simulink model "Core_Model_Controlled"  (R2023a)
settings: Solver=FixedStepAuto  StartTime=0.0  StopTime=Z  FixedStep=1/24  RelTol=1e-3
values from neighbouring files (symbols this model uses):
  c_eh = 0.85    [Model_Parameters.m]
  C_g = 1    [Model_Parameters.m]
  cc_e = -0.85    [Model_Parameters.m]
  id_a = 0.8*0.028*1.2    (= 0.02688)    [Model_Parameters.m]
  id_g = 0.8*0.072*1.2    (= 0.06912)    [Model_Parameters.m]
  id_l = 0.4*0.139*1.2    (= 0.06672)    [Model_Parameters.m]
  id_r = 0.4*0.428*1.2    (= 0.20544)    [Model_Parameters.m]
  id_z = 0.4*0.33*1.2    (= 0.1584)    [Model_Parameters.m]
  L_a = 0.25    [Model_Parameters.m]
  L_g = 0.1    [Model_Parameters.m]
  L_l = 0.2    [Model_Parameters.m]
  L_r = 0.05    [Model_Parameters.m]
  L_z = 0.08    [Model_Parameters.m]
  R_H2 = 0.05    [Model_Parameters.m]
  R_lh = 0.025    [Model_Parameters.m]
  R_ng = 0.025    [Model_Parameters.m]
  SF_MWh = SF_GWh*1e3    [Main_Script.m]
libraries: fl_lib x120, nesl_utility x93, ee_lib x36, slpidlib x1
(part 1 of 3)
settings Model: Creator=pienv  LastModifiedBy=pienv

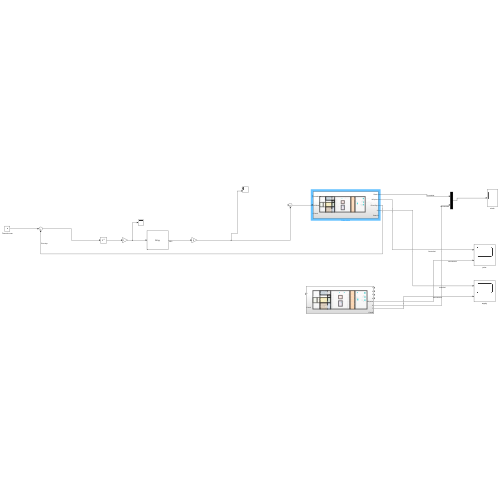
[thumbnail: Simulink's stored preview of the top-level diagram]
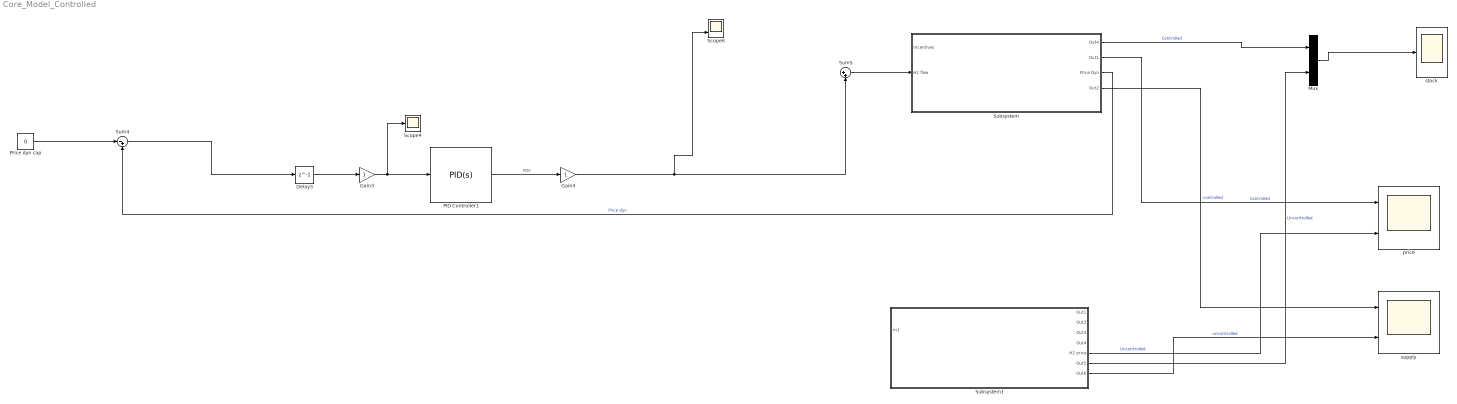
== system Core_Model_Controlled ==
  Delay3 : Delay  DelayLength=1
  Gain3 : Gain
  Gain4 : Gain
  Mux : Mux  Inputs=2
  PID Controller1 : slpidlib/PID Controller  Controller=PID  Form=Parallel  TimeDomain=Continuous-time  UseExternalTs=off  SampleTime=1/24  IntegratorMethod=Forward Euler  FilterMethod=Forward Euler  ControllerParametersSource=internal  P=20  I=4  UseKiTs=off  D=10  N=1  UseFilter=on  TunerSelectOption=Transfer Function Based (PID Tuner App)  InitialConditionSource=internal  InitialConditionForIntegrator=0  InitialConditionForFilter=0  DifferentiatorICPrevScaledInput=0  ExternalReset=none  TrackingMode=off  Kt=1  LimitOutput=off  SatLimitsSource=internal  UpperSaturationLimit=inf  LowerSaturationLimit=-inf  LinearizeAsGain=on  AntiWindupMode=none  Kb=1  LimitIntegrator=off  UpperIntegratorSaturationLimit=inf  LowerIntegratorSaturationLimit=-inf  POutMin=[]  POutMax=[]  IOutMin=[]  IOutMax=[]  DOutMin=[]  DOutMax=[]  NOutMin=[]  NOutMax=[]  SumOutMin=[]  SumOutMax=[]  SaturationOutMin=[]  SaturationOutMax=[]  PParamMin=[]  PParamMax=[]  IParamMin=[]  IParamMax=[]  DParamMin=[]  DParamMax=[]  NParamMin=[]  NParamMax=[]  KbParamMin=[]  KbParamMax=[]  KtParamMin=[]  KtParamMax=[]  KbOutMin=[]  KbOutMax=[]  KtOutMin=[]  KtOutMax=[]  IntegratorOutMin=[]  IntegratorOutMax=[]  FilterOutMin=[]  FilterOutMax=[]  SumI1OutMin=[]  SumI1OutMax=[]  SumI2OutMin=[]  SumI2OutMax=[]  SumI3OutMin=[]  SumI3OutMax=[]  SumI4OutMin=[]  SumI4OutMax=[]  SumDOutMin=[]  SumDOutMax=[]  DifferentiatorOutMin=[]  DifferentiatorOutMax=[]  FilterDiffOutCoefMin=[]  FilterDiffOutCoefMax=[]  ReciprocalOutMin=[]  ReciprocalOutMax=[]  SumDenOutMin=[]  SumDenOutMax=[]  SumNumOutMin=[]  SumNumOutMax=[]  DivideOutMin=[]  DivideOutMax=[]  UdiffTsProdOutMin=[]  UdiffTsProdOutMax=[]  NTsProdOutMin=[]  NTsProdOutMax=[]  UintegralTsProdOutMin=[]  UintegralTsProdOutMax=[]  UngainTsProdOutMin=[]  UngainTsProdOutMax=[]  ClampingZeroOutDataTypeStr=Inherit: Inherit via back propagation  ClampingZeroOutMin=[]  ClampingZeroOutMax=[]  FilterDenConstantOutDataTypeStr=Inherit: Inherit via back propagation  FilterDenConstantOutMin=[]  FilterDenConstantOutMax=[]  PCopyOutDataTypeStr=Inherit: Inherit via back propagation  PCopyOutMin=[]  PCopyOutMax=[]  NCopyOutDataTypeStr=Inherit: Inherit via back propagation  NCopyOutMin=[]  NCopyOutMax=[]  IntegratorContinuousStateAttributes=''  IntegratorStateMustResolveToSignalObject=off  IntegratorRTWStateStorageClass=Auto  FilterContinuousStateAttributes=''  FilterStateMustResolveToSignalObject=off  FilterRTWStateStorageClass=Auto  ParallelPVariant=InternalParameters  IdealPVariant=Disabled  IVariant=InternalParameters  DVariant=InternalParameters  IntegratorVariant=Continuous  SatVariant=Disabled  AWVariant=Passthrough  PCopyVariant=Disabled  TRVariant=Disabled  FdbkBlocksVariant=Forward  IdealPFdbkVariant=Disabled  SatFdbkVariant=Disabled  DerivativeFilterVariant=ContFilter  NVariant=InternalParameters  NCopyVariant=Disabled  FilterICVariant=InternalICsFilter  IntegratorICVariant=InternalICs  ExternalResetVariant=Disabled  TRSumVariant=Passthrough  SumFdbkVariant=Disabled  SumVariant=Sum_PID  TsampFilterVariant=InternalTs  TsampNgainVariant=Passthrough  TsampIntegralVariant=Disabled_SignalSpec  ExternalSaturationOutDataTypeStr=Inherit: Same as second input
  Price dyn cap : Constant  Value=0
  Scope4 : Scope
  Scope6 : Scope  NumInputPorts=2
  Subsystem : Subsystem
  Subsystem1 : Subsystem
  Sum4 : Sum  Inputs=|-+
  Sum5 : Sum  Inputs=|++
  price : Scope  NumInputPorts=2
  stock : Scope
  supply : Scope  NumInputPorts=2
  wires:
  Subsystem/2(Out1) -> price/1  "Controlled"
  Mux/1 -> stock/1
  Subsystem/1(Out4) -> Mux/1  "Controlled"
  Price dyn cap/1 -> Sum4/1
  Gain3/1 -> Scope4/1, PID Controller1/1
  Delay3/1 -> Gain3/1
  Sum4/1 -> Delay3/1
  PID Controller1/1 -> Gain4/1  "PDC"
  Subsystem/3(Price Dyn) -> Sum4/2  "Price dyn"
  Sum5/1 -> Subsystem/2(H2 flow)
  Gain4/1 -> Scope6/2, Sum5/2
  Subsystem1/5(H2 price) -> price/2  "Uncontrolled"
  Subsystem1/6(Out5) -> Mux/2  "Uncontrolled"
  Subsystem1/7(Out6) -> supply/2  "uncontrolled"
  Subsystem/4(Out2) -> supply/1  "controlled"

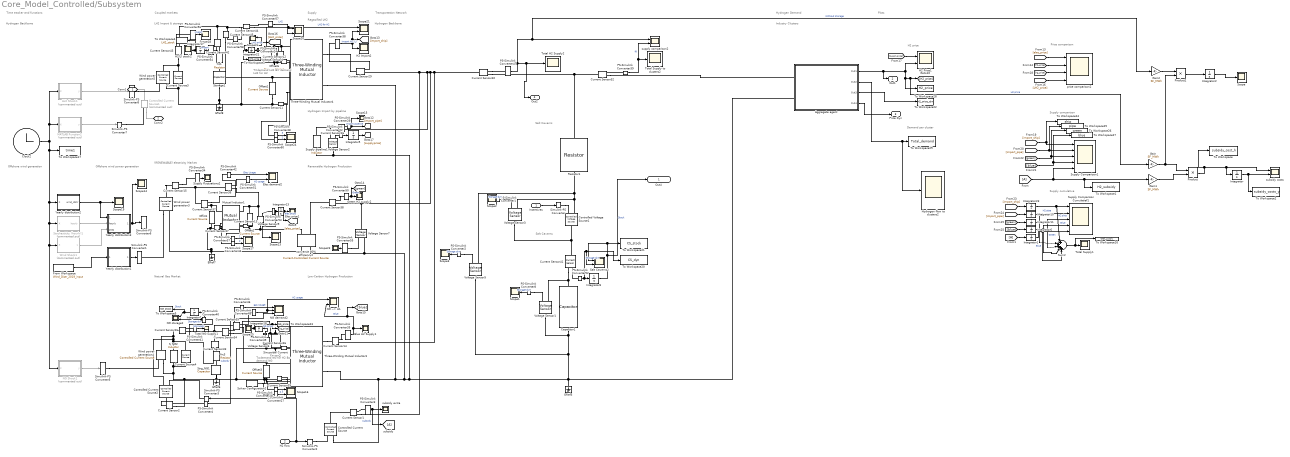
== system Core_Model_Controlled/Subsystem ==
  note: H2 price
  note: Supply cumulative
  note: Demand per cluster
  note: Renewable Hydrogen Production
  note: Offshore wind generation
  note: Hydrogen Import by pipeline
  note: Time tracker and functions
  note: Regasified LH2
  note: Hydrogen Backbone
  note: Hydrogen Backbone
  note: Coupled markets
  note: Supply comparison
  note: Salt Caverns
  note: Price comparison
  note: Transportation Network
  note: Plots
  note: Industry Clusters
  note: Hydrogen Demand
  note: Low-Carbon Hydrogen Production
  note: LH2 Import & storage
  note: T=demand LH2
      | B= demand LH2 for H2
  note: (RENEWABLE) electricity Market
  note: T=demand NG for H2
      | B= demand NG
  note: Supply
  note: Salt Caverns
  note: Offshore wind power generation
  note: Natural Gas Market
  Incentives : Inport
  H2 flow : Inport  Port=2
  Aggregate agent : Subsystem
  Blue H2 Supply1 : Scope
  Capacitor1 : fl_lib/Electrical/Electrical Elements/Capacitor  c=C_sc F  r=0 Ohm  g=0 1/Ohm  i_specify=on  i_priority=None  i=0.1 A  i_nominal_specify=off  i_nominal_unit=A  i_nominal_value=0.1  v_specify=off  v_priority=None  v=0 V  v_nominal_specify=off  v_nominal_unit=V  v_nominal_value=1  vc_specify=off  vc_priority=High  vc=0 V  vc_nominal_specify=off  vc_nominal_unit=V  vc_nominal_value=1
  Clock2 : Clock
      settings: Decimation=24
  Controlled Current Source : fl_lib/Electrical/Electrical Sources/Controlled Current Source
  Controlled Current Source1 : fl_lib/Electrical/Electrical Sources/Controlled Current Source  Commented=on
  Controlled Current Source2 : fl_lib/Electrical/Electrical Sources/Controlled Current Source
  Controlled Voltage Source1 : fl_lib/Electrical/Electrical Sources/Controlled Voltage Source
  Current Sensor{1..2,11..16,26,29,32..47} (26 alike) : fl_lib/Electrical/Electrical Sensors/Current Sensor
  Current Source3 : ee_lib/Sources/Current Source  dc_current=I_LH2 A  ac_current=0 A  ac_shift=0 rad  ac_frequency=60 Hz  noise_mode=ee.enum.sources.noise.Disabled  PSD=0 A^2/Hz  sample_time=1e-3 s  repeatability=ee.enum.sources.repeatability.NotRepeatable  user_seed=0  auto_seed=3890346746  i_specify=off  i_priority=None  i=0 A  i_nominal_specify=off  i_nominal_unit=A  i_nominal_value=1  v_specify=off  v_priority=None  v=0 V  v_nominal_specify=off  v_nominal_unit=V  v_nominal_value=1
  Current Source4 : ee_lib/Sources/Current Source  dc_current=v_sng A  ac_current=0 A  ac_shift=0 rad  ac_frequency=60 Hz  noise_mode=ee.enum.sources.noise.Disabled  PSD=0 A^2/Hz  sample_time=1e-3 s  repeatability=ee.enum.sources.repeatability.NotRepeatable  user_seed=0  auto_seed=545404223  i_specify=off  i_priority=None  i=0 A  i_nominal_specify=off  i_nominal_unit=A  i_nominal_value=1  v_specify=off  v_priority=None  v=0 V  v_nominal_specify=off  v_nominal_unit=V  v_nominal_value=1
  ERef{5..8} (4 alike) : fl_lib/Electrical/Electrical Elements/Electrical Reference
  Elec demand2 : Scope  NumInputPorts=2
  Elec price1 : Scope
  From : From
  From Workspace : FromWorkspace  VariableName=Wind_Distr_2019_input  OutDataTypeStr=double
  From1 : From
  Gain : Gain  Gain=SF_MWh
  Gain1 : Gain  Gain=SF_MWh
  Gain2 : Gain  Gain=SF_MWh
  Green H2 supply2 : Scope
  H2 Import2 : Scope
  H2 Price1 : Scope  NumInputPorts=2
  H2(L) stock2 : Scope
  Hydrogen flow to clusters2 : Scope
  Integrator{,1..2,5..8,10..11,13,17..18,21,23} (14 alike) : Integrator
  LH2 Shock1 : MATLAB Function  Commented=on  TreatAsAtomicUnit=on
  MATLAB Function2 : MATLAB Function  Commented=on  TreatAsAtomicUnit=on
  Mutual Inductor1 : fl_lib/Electrical/Electrical Elements/Mutual Inductor  L1=L_eh H  L2=L_e H  k=cc_e  i1_specify=off  i1_priority=High  i1=0 A  i1_nominal_specify=off  i1_nominal_unit=A  i1_nominal_value=1  i2_specify=off  i2_priority=High  i2=0 A  i2_nominal_specify=off  i2_nominal_unit=A  i2_nominal_value=1  v1_specify=off  v1_priority=None  v1=0 V  v1_nominal_specify=off  v1_nominal_unit=V  v1_nominal_value=1  v2_specify=off  v2_priority=None  v2=0 V  v2_nominal_specify=off  v2_nominal_unit=V  v2_nominal_value=1
      settings: InternalSimscapePortConfiguration="{\"Bottom\":[],\"Left\":[{\"id\":\"p1\",\"label\":\"1+\",\"type\":\"foundation.electrical.electrical\"},{\"id\":\"n1\",\"label\":\"1-\",\"type\":\"foundation.electrical.electrical\"}],\"Right\":[{\"id\":\"p2\",\"label\":\"2+\",\"type\":\"foundation.electrical.electrical\"},{\"id\":\"n2\",\"label\":\"2-\",\"type\":\"foundation.electrical.electrical\"}],\"Top\":[]}"
  NG --> H1 : Scope  NumInputPorts=2
  NG Shock1 : MATLAB Function  Commented=on  TreatAsAtomicUnit=on
  NG demand2 : Scope  NumInputPorts=3
  NG storage2 : Scope  NumInputPorts=2
  Offset1 : ee_lib/Sources/Current Source  dc_current=id_lh2h A  ac_current=0 A  ac_shift=0 rad  ac_frequency=0 Hz  noise_mode=0  PSD=0 A^2/Hz  sample_time=1e-3 s  repeatability=1  user_seed=0  auto_seed=3922919431  i_specify=off  i_priority=None  i=0 A  i_nominal_specify=off  i_nominal_unit=A  i_nominal_value=1  v_specify=off  v_priority=None  v=0 V  v_nominal_specify=off  v_nominal_unit=V  v_nominal_value=1
  Offset2 : ee_lib/Sources/Current Source  dc_current=id_eh A  ac_current=0 A  ac_shift=0 rad  ac_frequency=0 Hz  noise_mode=0  PSD=0 A^2/Hz  sample_time=1e-3 s  repeatability=1  user_seed=0  auto_seed=2715962282  i_specify=off  i_priority=None  i=0 A  i_nominal_specify=off  i_nominal_unit=A  i_nominal_value=1  v_specify=off  v_priority=None  v=0 V  v_nominal_specify=off  v_nominal_unit=V  v_nominal_value=1
  Offset3 : ee_lib/Sources/Current Source  dc_current=id_ngh A  ac_current=0 A  ac_shift=0 rad  ac_frequency=0 Hz  noise_mode=0  PSD=0 A^2/Hz  sample_time=1e-3 s  repeatability=1  user_seed=0  auto_seed=418932850  i_specify=off  i_priority=None  i=0 A  i_nominal_specify=off  i_nominal_unit=A  i_nominal_value=1  v_specify=off  v_priority=None  v=0 V  v_nominal_specify=off  v_nominal_unit=V  v_nominal_value=1
  Offset6 : ee_lib/Sources/Current Source  dc_current=id_lh2 A  ac_current=0 A  ac_shift=0 rad  ac_frequency=0 Hz  noise_mode=0  PSD=0 A^2/Hz  sample_time=1e-3 s  repeatability=1  user_seed=0  auto_seed=1196140742  i_specify=off  i_priority=None  i=0 A  i_nominal_specify=off  i_nominal_unit=A  i_nominal_value=1  v_specify=off  v_priority=None  v=0 V  v_nominal_specify=off  v_nominal_unit=V  v_nominal_value=1
  Offst1 : ee_lib/Sources/Current Source  dc_current=id_e A  ac_current=0 A  ac_shift=0 rad  ac_frequency=0 Hz  noise_mode=0  PSD=0 A^2/Hz  sample_time=1e-3 s  repeatability=1  user_seed=0  auto_seed=2348838240  i_specify=off  i_priority=None  i=0 A  i_nominal_specify=off  i_nominal_unit=A  i_nominal_value=1  v_specify=off  v_priority=None  v=0 V  v_nominal_specify=off  v_nominal_unit=V  v_nominal_value=1
  PS-Simulink Converter{1..4,8,22,24,27..29,34..35,37..42,44..56,60} (32 alike) : nesl_utility/PS-Simulink Converter  PhysicalDomain=network_engine_domain  SubClassName=ps_output  LeftPortType=input  RightPortType=output  PseudoPeriodic=off  Frequencies=[]  VectorFormat=1-D array  Unit=1  AffineConversion=off
  PS-Simulink Converter57 : nesl_utility/PS-Simulink Converter  PhysicalDomain=network_engine_domain  SubClassName=ps_output  LeftPortType=input  RightPortType=output  PseudoPeriodic=off  Frequencies=[]  VectorFormat=inherit  Unit=inherit  AffineConversion=off
  PS-Simulink Converter58 : nesl_utility/PS-Simulink Converter  PhysicalDomain=network_engine_domain  SubClassName=ps_output  LeftPortType=input  RightPortType=output  PseudoPeriodic=off  Frequencies=[]  VectorFormat=inherit  Unit=inherit  AffineConversion=off
  Product : Product
  Product1 : Product
  Resistor1 : fl_lib/Electrical/Electrical Elements/Resistor  R=R_H2 Ohm  i_specify=off  i_priority=None  i=0 A  i_nominal_specify=off  i_nominal_unit=A  i_nominal_value=1  v_specify=off  v_priority=None  v=0 V  v_nominal_specify=off  v_nominal_unit=V  v_nominal_value=1
  S_NG2 : ee_lib/Passive/Inductor  l=L_sng H  enable_L_tol=ee.enum.toleranceApplication.none  L_tol=20  tol_distribution=ee.enum.toleranceDistribution.uniform  nSigma=4  r=0 Ohm  g=0 1/Ohm  enable_operating_limits=ee.enum.enable.no  operating_limit_action=ee.enum.passive.reportOpLim.warn  max_working_current=1 A  power_rating=1 W  enable_faults=ee.enum.enable.no  fault_action=simscape.enum.assert.action.none  lambdaPercent=50  k_faulted=0.9999  turnsShort=ee.enum.passive.inductor.turnsShortOption.no  openCct=ee.enum.enable.no  groundShort=ee.enum.passive.inductor.groundShortOption.no  groundShortG=0 1/Ohm  tau_fault=1e-3 s  fault_trigger=ee.enum.faults.faultTrigger.temporal  t_fault=1 s  max_permissible_voltage=100 V  n_fail_on_voltage=1  max_permissible_current=1 A  t_fail_on_current=1 s  i_L_specify=off  i_L_priority=High  i_L=0 A  i_L_nominal_specify=off  i_L_nominal_unit=A  i_L_nominal_value=1
  Salt Caverns2 : Scope  NumInputPorts=2
  Scope{,1..3,13..15,18..19,23,25} (11 alike) : Scope
  Scope{16..17,20..22,24} (6 alike) : Scope  NumInputPorts=2
  Simulink-PS Converter{,2..3,5,7..8} (6 alike) : nesl_utility/Simulink-PS Converter  PhysicalDomain=network_engine_domain  SubClassName=ps_input  LeftPortType=input  RightPortType=output  PseudoPeriodic=off  Frequencies=[]  NoiseDistribution=none  NoiseParameters=[]  Unit=1  AffineConversion=off  FilteringAndDerivatives=provide  SimscapeFilterOrder=1  InputFilterTimeConstant=0.001  UdotUserProvided=0
  Simulink-PS Converter1 : nesl_utility/Simulink-PS Converter  PhysicalDomain=network_engine_domain  SubClassName=ps_input  LeftPortType=input  RightPortType=output  PseudoPeriodic=off  Frequencies=[]  NoiseDistribution=none  NoiseParameters=[]  Unit=1  AffineConversion=off  FilteringAndDerivatives=filter  SimscapeFilterOrder=2  InputFilterTimeConstant=0.001  UdotUserProvided=0
  Simulink-PS Converter6 : nesl_utility/Simulink-PS Converter  PhysicalDomain=network_engine_domain  SubClassName=ps_input  LeftPortType=input  RightPortType=output  PseudoPeriodic=off  Frequencies=[]  NoiseDistribution=none  NoiseParameters=[]  Unit=1  AffineConversion=off  FilteringAndDerivatives=filter  SimscapeFilterOrder=2  InputFilterTimeConstant=0.001  UdotUserProvided=0
  Sinusoidal Current Source2 : ee_lib/Additional Components/SPICE Sources/Sinusoidal Current Source  IO=id_ng_IO A  IA=id_ng_IA A  FREQ=id_ng_FREQ Hz  TD=id_ng_TD s  DF=0 1/s  Gmin_param=ee.enum.gminParam.yes
      settings: InternalSimscapePortConfiguration="{\"Bottom\":[],\"Left\":[{\"id\":\"p\",\"label\":\"+\",\"type\":\"foundation.electrical.electrical\"}],\"Right\":[{\"id\":\"n\",\"label\":\"-\",\"type\":\"foundation.electrical.electrical\"}],\"Top\":[]}"
  Solver Configuration2 : nesl_utility/Solver Configuration  PhysicalDomain=network_engine_domain  SubClassName=solver  LeftPortType=input  RightPortType=generic  Tones=[]  Harmonics=[]  SimulateNoise=off  Profile=off  UseLocalSampling=off  EnableSwitchedLinearOptims=on  FrequencyDomain=off  UseCCode=off  RelTol=0.001  AbsTol=0.001  MinStep=1e-09  ToWorkspace=off  RevertToSquareIcSolve=off  NumHomotopyIterations=100  PhasorMode=off  PhasorModeNumHarmonics=1  ConsistencySolver=NEWTON_XTOL_AFTER_FTOL  IndexReductionMethod=DerivativeReplacement  DoDC=off  ResidualTolerance=1e-09  ConsistencyTolSource=LOCAL  ConsistencyAbsTol=0.001  ConsistencyRelTol=0.001  ConsistencyTolFactor=0.001  UseLocalSolver=off  LocalSolverChoice=NE_BACKWARD_EULER_ADVANCER  ResolveIndetEquations=on  FunctionEvalNumThread=1  LocalSolverSampleTime=0.001  DoFixedCost=off  MaxNonlinIter=3  MaxModeIter=2  ComputeImpulses=off  ImpulseIterations=2  LinearAlgebra=auto  LinearAlgebraNumThread=0  EquationFormulation=NE_TIME_EF  DelaysMemoryBudget=1024  AutomaticFiltering=off  FilteringTimeConstant=0.0001  PartitionStorageMethod=AS_NEEDED  PartitionMemoryBudget=1024  PartitionMethod=ROBUST
  Stochasticity (hourly)1 : MATLAB Function  Commented=on  TreatAsAtomicUnit=on
  Storage1 : fl_lib/Electrical/Electrical Elements/Capacitor  c=C_lh F  r=0 Ohm  g=0 1/Ohm  i_specify=off  i_priority=None  i=0 A  i_nominal_specify=off  i_nominal_unit=A  i_nominal_value=1  v_specify=off  v_priority=None  v=0 V  v_nominal_specify=off  v_nominal_unit=V  v_nominal_value=1  vc_specify=off  vc_priority=High  vc=0 V  vc_nominal_specify=off  vc_nominal_unit=V  vc_nominal_value=1
  Strg_NG1 : fl_lib/Electrical/Electrical Elements/Capacitor  c=C_ng F  r=0 Ohm  g=0 1/Ohm  i_specify=off  i_priority=None  i=0 A  i_nominal_specify=off  i_nominal_unit=A  i_nominal_value=1  v_specify=off  v_priority=None  v=0 V  v_nominal_specify=off  v_nominal_unit=V  v_nominal_value=1  vc_specify=off  vc_priority=High  vc=0 V  vc_nominal_specify=off  vc_nominal_unit=V  vc_nominal_value=100
  Sum2 : Sum  Inputs=|+++++
  Supply pipeline1 : ee_lib/Passive/Inductor  l=L_i H  enable_L_tol=ee.enum.toleranceApplication.none  L_tol=20  tol_distribution=ee.enum.toleranceDistribution.uniform  nSigma=4  r=0 Ohm  g=0 1/Ohm  enable_operating_limits=ee.enum.enable.no  operating_limit_action=ee.enum.passive.reportOpLim.warn  max_working_current=1 A  power_rating=1 W  enable_faults=ee.enum.enable.no  fault_action=simscape.enum.assert.action.none  lambdaPercent=50  k_faulted=0.9999  turnsShort=ee.enum.passive.inductor.turnsShortOption.no  openCct=ee.enum.enable.no  groundShort=ee.enum.passive.inductor.groundShortOption.no  groundShortG=0 1/Ohm  tau_fault=1e-3 s  fault_trigger=ee.enum.faults.faultTrigger.temporal  t_fault=1 s  max_permissible_voltage=100 V  n_fail_on_voltage=1  max_permissible_current=1 A  t_fail_on_current=1 s  i_L_specify=off  i_L_priority=High  i_L=0 A  i_L_nominal_specify=off  i_L_nominal_unit=A  i_L_nominal_value=1
  Supply Comparison Cumulatief1 : Scope  NumInputPorts=5
  Supply Comparison1 : Scope  NumInputPorts=5
  Supply fluctuations2 : Scope
  Three-Winding Mutual Inductor3 : ee_lib/Passive/Transformers/Three-Winding Mutual Inductor  L1=L_sbh H  L2=L_ngh H  L3=L_ng H  K12=c_ng12  K13=c_ng13  K23=c_ng23  IC_given=1  IC1=0 A  IC2=0 A  IC3=0 A
      settings: LogSimulationData=on  InternalSimscapePortConfiguration="{\"Bottom\":[],\"Left\":[{\"id\":\"p1\",\"label\":\"1+\",\"type\":\"foundation.electrical.electrical\"},{\"id\":\"n1\",\"label\":\"1-\",\"type\":\"foundation.electrical.electrical\"}],\"Right\":[{\"id\":\"p2\",\"label\":\"2+\",\"type\":\"foundation.electrical.electrical\"},{\"id\":\"n2\",\"label\":\"2-\",\"type\":\"foundation.electrical.electrical\"},{\"id\":\"p3\",\"label\":\"3+\",\"type\":\"foundation.electrical.electrical\"},{\"id\":\"n3\",\"label\":\"3-\",\"type\":\"foundation.electrical.electrical\"}],\"Top\":[]}"
  Three-Winding Mutual Inductor4 : ee_lib/Passive/Transformers/Three-Winding Mutual Inductor  L1=L_sih H  L2=L_lh2h H  L3=L_lh2 H  K12=c_lh212  K13=c_lh213  K23=c_lh223  IC_given=1  IC1=0 A  IC2=0 A  IC3=0 A
      settings: LogSimulationData=on  InternalSimscapePortConfiguration="{\"Bottom\":[],\"Left\":[{\"id\":\"p1\",\"label\":\"1+\",\"type\":\"foundation.electrical.electrical\"},{\"id\":\"n1\",\"label\":\"1-\",\"type\":\"foundation.electrical.electrical\"}],\"Right\":[{\"id\":\"p2\",\"label\":\"2+\",\"type\":\"foundation.electrical.electrical\"},{\"id\":\"n2\",\"label\":\"2-\",\"type\":\"foundation.electrical.electrical\"},{\"id\":\"p3\",\"label\":\"3+\",\"type\":\"foundation.electrical.electrical\"},{\"id\":\"n3\",\"label\":\"3-\",\"type\":\"foundation.electrical.electrical\"}],\"Top\":[]}"
  To Workspace : ToWorkspace  VariableName=subsidy_cost_h  SampleTime=-1
  To Workspace1 : ToWorkspace  VariableName=H2_subsidy  SampleTime=-1
  To Workspace16 : ToWorkspace  VariableName=total_supply  SampleTime=-1
  To Workspace17 : ToWorkspace  VariableName=time1  SampleTime=-1
  To Workspace2 : ToWorkspace  VariableName=subsidy_costs_y  SampleTime=-1
  To Workspace20 : ToWorkspace  VariableName=CS_dyn  SampleTime=-1
      settings: Save2DSignal=2-D array (concatenate along first dimension)
  To Workspace21 : ToWorkspace  VariableName=CS_stock  SampleTime=-1
  To Workspace22 : ToWorkspace  VariableName=H2_price_dyn  SampleTime=-1
      settings: Save2DSignal=2-D array (concatenate along first dimension)
  To Workspace23 : ToWorkspace  VariableName=NG_price  SampleTime=-1
      settings: Save2DSignal=2-D array (concatenate along first dimension)
  To Workspace24 : ToWorkspace  VariableName=ship  SampleTime=-1
  To Workspace25 : ToWorkspace  VariableName=pipe  SampleTime=-1
  To Workspace26 : ToWorkspace  VariableName=green  SampleTime=-1
  To Workspace27 : ToWorkspace  VariableName=blue  SampleTime=-1
  To Workspace28 : ToWorkspace  VariableName=H2_price  SampleTime=-1
  To Workspace29 : ToWorkspace  VariableName=Total_demand  SampleTime=-1
      settings: Save2DSignal=2-D array (concatenate along first dimension)
  To Workspace3 : ToWorkspace  VariableName=LH2_price  SampleTime=-1
  To Workspace4 : ToWorkspace  VariableName=LH2_stock  SampleTime=-1
  To Workspace5 : ToWorkspace  VariableName=NG_stock  SampleTime=-1
  Total H2 Supply2 : Scope
  Total NG Supply1 : Scope
  Total Supply to clusters2 : Scope
  Total Supply1 : Scope
  Voltage Sensor{1..7,9} (8 alike) : fl_lib/Electrical/Electrical Sensors/Voltage Sensor
  Wind Shock1 : MATLAB Function  Commented=on  TreatAsAtomicUnit=on
  Wind power generation3 : fl_lib/Electrical/Electrical Sources/Controlled Current Source
  Wind power generation4 : fl_lib/Electrical/Electrical Sources/Controlled Current Source
  Wind power generation5 : fl_lib/Electrical/Electrical Sources/Controlled Current Source
  Yearly distribution1 : MATLAB Function  TreatAsAtomicUnit=on
  Yearly distribution2 : MATLAB Function  TreatAsAtomicUnit=on
  Yearly distribution3 : MATLAB Function  TreatAsAtomicUnit=on
  conversie 80% efficiency2 : fl_lib/Electrical/Electrical Sources/Current-Controlled Current Source  K=c_eh  i1_specify=off  i1_priority=None  i1=0 A  i1_nominal_specify=off  i1_nominal_unit=A  i1_nominal_value=1  i2_specify=off  i2_priority=None  i2=0 A  i2_nominal_specify=off  i2_nominal_unit=A  i2_nominal_value=1
      settings: InternalSimscapePortConfiguration="{\"Bottom\":[],\"Left\":[{\"id\":\"p1\",\"label\":\"+\",\"type\":\"foundation.electrical.electrical\"},{\"id\":\"head\",\"label\":\"\",\"type\":\"foundation.electrical.electrical\"}],\"Right\":[{\"id\":\"n1\",\"label\":\"-\",\"type\":\"foundation.electrical.electrical\"},{\"id\":\"tail\",\"label\":\"\",\"type\":\"foundation.electrical.electrical\"}],\"Top\":[]}"
  frc1 : fl_lib/Electrical/Electrical Elements/Resistor  R=R_lh Ohm  i_specify=off  i_priority=High  i=0 A  i_nominal_specify=off  i_nominal_unit=A  i_nominal_value=1  v_specify=off  v_priority=High  v=0 V  v_nominal_specify=off  v_nominal_unit=V  v_nominal_value=1
      settings: AttributesFormatString=%<R> %<R_unit>
  frc3 : fl_lib/Electrical/Electrical Elements/Resistor  R=R_ng Ohm  i_specify=off  i_priority=High  i=0 A  i_nominal_specify=off  i_nominal_unit=A  i_nominal_value=1  v_specify=off  v_priority=High  v=0 V  v_nominal_specify=off  v_nominal_unit=V  v_nominal_value=1
      settings: AttributesFormatString=%<R> %<R_unit>
  price comparison2 : Scope  NumInputPorts=4
  subsidy : Goto
  subsidy costs : Scope  NumInputPorts=2
  subsidy extra : Scope
  supply comparison2 : Scope  NumInputPorts=2
  Conn1 : PMIOPort  Side=Left
  Conn2 : PMIOPort  Port=2  Side=Right
  Out4 : Outport
  Out1 : Outport  Port=2
  Price Dyn : Outport  Port=3
  Out2 : Outport  Port=4
  wires:
  Integrator10/1 -> Supply Comparison Cumulatief1/2, Sum2/2  "H2 pipe"
  PS-Simulink Converter39/1 -> Total Supply to clusters2/1, supply comparison2/2  "fd"
  [import_ship] -> Integrator23/1
  Integrator11/1 -> Supply Comparison Cumulatief1/3, Sum2/3  "Green"
  PS-Simulink Converter38/1 -> Scope21/2, [import_ship], H2 Import2/1  "Import H2 (L)"
  Clock2/1 -> LH2 Shock1/1(X), MATLAB Function2/1(X), NG Shock1/1(X), Wind Shock1/1(X), Stochasticity (hourly)1/1(X), Yearly distribution2/1(X), To Workspace17/1
  PS-Simulink Converter52/1 -> To Workspace20/1, Salt Caverns2/2, Integrator8/1  "Storage dyn"
  PS-Simulink Converter29/1 -> Scope15/1, [import_pipe]  "import pipeline"
  PS-Simulink Converter48/1 -> Scope24/1  "3"
  LH2 Shock1/1(y) -> Simulink-PS Converter8/1
  Yearly distribution3/1(current) -> Scope14/1, Simulink-PS Converter6/1
  PS-Simulink Converter55/1 -> Scope23/1
  Aggregate agent/2(Out2) -> Hydrogen flow to clusters2/1, To Workspace29/1
  PS-Simulink Converter24/1 -> Integrator21/1
  Integrator18/1 -> [ng_price], To Workspace23/1, Scope25/1  "NG price"
  Stochasticity (hourly)1/1(hourly) -> Yearly distribution3/2(hourly)
  PS-Simulink Converter42/1 -> Elec demand2/1  "Elec Usage"
  PS-Simulink Converter27/1 -> Scope16/1  "3"
  [H2_price] -> price comparison2/2
  Wind Shock1/1(y) -> Yearly distribution3/3(step)
  Integrator7/1 -> To Workspace5/1, NG storage2/1  "Stock"
  PS-Simulink Converter37/1 -> Scope17/1  "1"
  PS-Simulink Converter54/1 -> Integrator17/1  "Import"
  PS-Simulink Converter60/1 -> Scope24/2  "2"
  PS-Simulink Converter44/1 -> Scope17/2  "2"
  Sum2/1 -> To Workspace16/1, Total Supply1/1
  NG Shock1/1(y) -> Simulink-PS Converter5/1
  PS-Simulink Converter35/1 -> [blue], NG --> H1/2, Blue H2 Supply1/1  "Blue"
  PS-Simulink Converter57/1 -> Scope20/2  "LH2"
  Integrator6/1 -> Supply Comparison Cumulatief1/4, Sum2/4  "Blue"
  Aggregate agent/1(Out1) -> Out1/1, To Workspace28/1, Gain/1, [H2_price], H2 Price1/2  "H2 price"
  Integrator21/1 -> To Workspace3/1, Scope22/1, [LH2_price]  "LH2 price"
  [blue] -> To Workspace27/1, Supply Comparison1/4
  Integrator8/1 -> Out4/1, To Workspace21/1, Salt Caverns2/1  "Stock"
  PS-Simulink Converter50/1 -> [green], Green H2 supply2/1  "Green"
  [import_pipe] -> To Workspace25/1, Supply Comparison1/2
  PS-Simulink Converter40/1 -> Integrator7/1, NG storage2/2  "Storage dyn"
  PS-Simulink Converter53/1 -> Scope13/1, Integrator13/1
  PS-Simulink Converter58/1 -> Scope21/1, Scope20/1  "LH2 for H2"
  PS-Simulink Converter45/1 -> NG --> H1/1, NG demand2/2  "H2 usage"
  [elec_price] -> price comparison2/1
  PS-Simulink Converter51/1 -> Elec demand2/2  "H2 usage"
  Integrator13/1 -> [elec_price], Elec price1/1  "elec price"
  [ng_price] -> price comparison2/3
  Yearly distribution2/1(wind_distr) -> Yearly distribution3/1(wind_distr), Scope19/1
  Integrator23/1 -> Supply Comparison Cumulatief1/1, Sum2/1  "H2 ship"
  PS-Simulink Converter56/1 -> Scope18/1  "Import"
  [green] -> To Workspace26/1, Supply Comparison1/3
  [import_ship] -> To Workspace24/1, Supply Comparison1/1
  PS-Simulink Converter41/1 -> Total NG Supply1/1  "NG supply"
  [green] -> Integrator11/1
  Integrator17/1 -> To Workspace4/1, H2(L) stock2/1
  Integrator5/1 -> [supplyprice]
  PS-Simulink Converter47/1 -> Gain2/1, supply comparison2/1, Out2/1, Total H2 Supply2/1  "Without storage"
  [blue] -> Integrator6/1
  [supplyprice] -> H2 Price1/1
  PS-Simulink Converter49/1 -> Integrator18/1
  [import_pipe] -> Integrator10/1
  PS-Simulink Converter22/1 -> Integrator5/1
  MATLAB Function2/1(y) -> Simulink-PS Converter7/1
  PS-Simulink Converter34/1 -> Supply fluctuations2/1
  Aggregate agent/3(Out3) -> To Workspace22/1
  [LH2_price] -> price comparison2/4
  PS-Simulink Converter28/1 -> Scope16/2  "2"
  PS-Simulink Converter46/1 -> NG demand2/1  "gas Usage"
  Incentives/1 -> Simulink-PS Converter/1
  From Workspace/1 -> Yearly distribution1/1(wind_distr)
  Yearly distribution1/1(current) -> Simulink-PS Converter1/1
  PS-Simulink Converter8/1 -> Scope1/1  "Storage dyn"
  PS-Simulink Converter1/1 -> Scope2/1  "Storage dyn"
  PS-Simulink Converter2/1 -> Scope3/1  "Storage dyn"
  H2 flow/1 -> Simulink-PS Converter3/1, Simulink-PS Converter2/1
  PS-Simulink Converter3/1 -> subsidy/1, subsidy extra/1  "subsidy"
  From/1 -> To Workspace1/1, Gain1/1, Supply Comparison1/5
  Product/1 -> To Workspace/1, Integrator/1, subsidy costs/1
  Integrator/1 -> To Workspace2/1, subsidy costs/2
  Gain/1 -> Product1/2, Product/1
  Gain1/1 -> Product/2
  From1/1 -> Integrator1/1
  Integrator1/1 -> Sum2/5, Supply Comparison Cumulatief1/5  "Blue"
  PS-Simulink Converter4/1 -> NG demand2/3  "subsidy"
  Aggregate agent/4(Out4) -> Price Dyn/1
  Gain2/1 -> Product1/1
  Product1/1 -> Integrator2/1
  Integrator2/1 -> Scope/1
  connections:
  Current Sensor44/LConn1 -- Current Sensor45/LConn1 -- Current Sensor42/LConn1 -- Current Sensor43/RConn2
  Current Sensor40/RConn1 -- PS-Simulink Converter47/LConn1
  Voltage Sensor5/LConn1 -- Voltage Sensor1/LConn1 -- Capacitor1/LConn1 -- Aggregate agent/LConn2 -- ERef5/LConn1 -- Supply pipeline1/LConn1 -- Voltage Sensor2/LConn1 -- conversie 80% efficiency2/RConn2 -- Voltage Sensor7/RConn2 -- Three-Winding Mutual Inductor4/LConn1 -- Controlled Current Source/RConn2 -- Three-Winding Mutual Inductor3/LConn1
  PS-Simulink Converter45/LConn1 -- Current Sensor35/RConn1
  Current Sensor32/RConn2 -- Aggregate agent/LConn1
  PS-Simulink Converter39/LConn1 -- Current Sensor32/RConn1
  frc1/RConn1 -- Current Sensor42/RConn2
  Offset3/RConn1 -- Three-Winding Mutual Inductor3/RConn2 -- Current Sensor35/RConn2
  Supply pipeline1/RConn1 -- Voltage Sensor2/RConn2 -- Current Sensor16/LConn1
  Three-Winding Mutual Inductor3/RConn4 -- Sinusoidal Current Source2/LConn1 -- Voltage Sensor6/RConn2 -- Current Sensor34/RConn2
  PS-Simulink Converter35/LConn1 -- Current Sensor14/RConn1
  Three-Winding Mutual Inductor4/LConn2 -- Current Sensor29/LConn1
  Current Sensor36/RConn2 -- Mutual Inductor1/LConn2 -- Offset2/RConn1 -- Voltage Sensor9/RConn2
  PS-Simulink Converter38/LConn1 -- Current Sensor29/RConn1
  PS-Simulink Converter41/LConn1 -- Current Sensor26/RConn1
  PS-Simulink Converter28/LConn1 -- Current Sensor39/RConn1
  PS-Simulink Converter50/LConn1 -- Current Sensor38/RConn1
  Simulink-PS Converter7/RConn1 -- Controlled Current Source1/RConn1
  Current Sensor15/RConn1 -- PS-Simulink Converter34/LConn1
  Current Sensor38/LConn1 -- conversie 80% efficiency2/LConn2
  Offset2/LConn1 -- Current Sensor13/LConn1 -- conversie 80% efficiency2/LConn1 -- Voltage Sensor9/LConn1
  PS-Simulink Converter22/LConn1 -- Voltage Sensor2/RConn1
  PS-Simulink Converter24/LConn1 -- Voltage Sensor4/RConn1
  Current Sensor11/LConn1 -- Offset1/LConn1 -- ERef8/LConn1 -- Storage1/LConn1 -- Wind power generation5/RConn2 -- Current Source3/RConn1 -- Voltage Sensor4/LConn1 -- Current Sensor12/LConn1 -- Offset6/LConn1
  Offset6/RConn1 -- Current Sensor44/RConn2 -- Three-Winding Mutual Inductor4/RConn4 -- Voltage Sensor4/RConn2
  PS-Simulink Converter58/LConn1 -- Current Sensor45/RConn1
  conversie 80% efficiency2/RConn1 -- Offst1/LConn1 -- Current Sensor47/LConn1 -- ERef7/LConn1 -- Wind power generation3/RConn2
  Current Sensor26/RConn2 -- Current Sensor35/LConn1 -- Current Sensor34/LConn1 -- Current Sensor33/LConn1
  Offset3/LConn1 -- Current Sensor39/LConn1 -- Solver Configuration2/RConn1 -- Sinusoidal Current Source2/RConn1 -- Current Sensor46/LConn1 -- Voltage Sensor6/LConn1 -- Current Sensor2/RConn2 -- Wind power generation4/RConn2 -- Current Source4/RConn1 -- S_NG2/LConn1 -- Strg_NG1/LConn1 -- ERef6/LConn1
  frc3/LConn1 -- Strg_NG1/RConn1
  Controlled Current Source1/LConn1 -- Conn1/RConn1
  Current Sensor43/LConn1 -- Wind power generation5/LConn1 -- Current Source3/LConn1
  Current Sensor39/RConn2 -- Three-Winding Mutual Inductor3/RConn1
  Current Sensor37/LConn1 -- Current Sensor15/RConn2 -- Current Sensor36/LConn1
  Controlled Current Source/LConn1 -- Current Sensor1/LConn1
  S_NG2/RConn1 -- Current Source4/LConn1 -- Controlled Current Source2/RConn2 -- Wind power generation4/LConn1 -- Current Sensor26/LConn1
  PS-Simulink Converter53/LConn1 -- Voltage Sensor9/RConn1
  Offset1/RConn1 -- Three-Winding Mutual Inductor4/RConn2 -- Current Sensor45/RConn2
  Current Sensor40/RConn2 -- Current Sensor32/LConn1 -- Resistor1/RConn1
  Controlled Current Source1/RConn2 -- Conn2/RConn1
  Current Sensor13/RConn1 -- PS-Simulink Converter37/LConn1
  PS-Simulink Converter60/LConn1 -- Current Sensor11/RConn1
  PS-Simulink Converter57/LConn1 -- Current Sensor44/RConn1
  PS-Simulink Converter52/LConn1 -- Current Sensor41/RConn1
  Current Sensor15/LConn1 -- Wind power generation3/LConn1
  Storage1/RConn1 -- frc1/LConn1
  PS-Simulink Converter49/LConn1 -- Voltage Sensor6/RConn1
  PS-Simulink Converter51/LConn1 -- Current Sensor36/RConn1
  Current Sensor33/RConn1 -- PS-Simulink Converter40/LConn1
  Mutual Inductor1/RConn2 -- Offst1/RConn1 -- Current Sensor37/RConn2
  PS-Simulink Converter27/LConn1 -- Current Sensor46/RConn1
  PS-Simulink Converter56/LConn1 -- Current Sensor43/RConn1
  PS-Simulink Converter46/LConn1 -- Current Sensor34/RConn1
  Current Sensor12/RConn2 -- Three-Winding Mutual Inductor4/RConn3
  Three-Winding Mutual Inductor3/LConn2 -- Current Sensor14/LConn1
  Current Sensor47/RConn2 -- Mutual Inductor1/RConn1
  PS-Simulink Converter55/LConn1 -- Voltage Sensor7/RConn1
  Three-Winding Mutual Inductor3/RConn3 -- Current Sensor46/RConn2
  Current Sensor33/RConn2 -- frc3/RConn1
  Current Sensor41/RConn2 -- Capacitor1/RConn1 -- Voltage Sensor1/RConn2
  Simulink-PS Converter8/RConn1 -- Wind power generation5/RConn1
  PS-Simulink Converter48/LConn1 -- Current Sensor12/RConn1
  Current Sensor37/RConn1 -- PS-Simulink Converter42/LConn1
  PS-Simulink Converter29/LConn1 -- Current Sensor16/RConn1
  Simulink-PS Converter5/RConn1 -- Wind power generation4/RConn1
  PS-Simulink Converter54/LConn1 -- Current Sensor42/RConn1
  Current Sensor13/RConn2 -- Mutual Inductor1/LConn1
  Three-Winding Mutual Inductor4/RConn1 -- Current Sensor11/RConn2
  Current Sensor47/RConn1 -- PS-Simulink Converter44/LConn1
  Simulink-PS Converter/RConn1 -- Controlled Voltage Source1/RConn1
  Voltage Sensor3/RConn2 -- Controlled Voltage Source1/RConn2 -- Resistor1/LConn1 -- Voltage Sensor5/RConn2
  Voltage Sensor3/LConn1 -- Current Sensor41/LConn1 -- Controlled Voltage Source1/LConn1
  PS-Simulink Converter8/LConn1 -- Voltage Sensor1/RConn1
  PS-Simulink Converter1/LConn1 -- Voltage Sensor3/RConn1
  PS-Simulink Converter2/LConn1 -- Voltage Sensor5/RConn1
  Simulink-PS Converter2/RConn1 -- Controlled Current Source/RConn1
  Current Sensor1/RConn2 -- Current Sensor40/LConn1 -- Current Sensor14/RConn2 -- Current Sensor38/RConn2 -- Voltage Sensor7/LConn1 -- Current Sensor16/RConn2 -- Current Sensor29/RConn2
  PS-Simulink Converter3/LConn1 -- Current Sensor1/RConn1
  Wind power generation3/RConn1 -- Simulink-PS Converter1/RConn1
  Simulink-PS Converter3/RConn1 -- Controlled Current Source2/RConn1
  Controlled Current Source2/LConn1 -- Current Sensor2/LConn1
  PS-Simulink Converter4/LConn1 -- Current Sensor2/RConn1
